simulink model "D_Latch"  (R2020a)
settings: Solver=VariableStepAuto  StartTime=0.0  StopTime=10.0  RelTol=1e-3
settings Model: Creator=ashwin  LastModifiedBy=ashwin

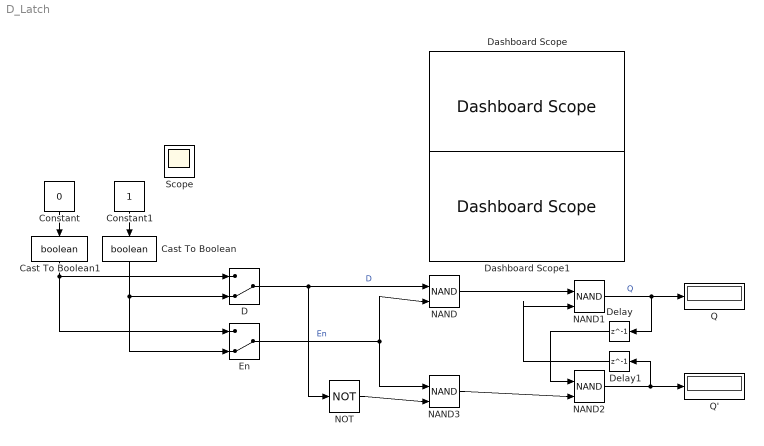
== system D_Latch ==
  Cast To Boolean : DataTypeConversion  OutDataTypeStr=boolean
  Cast To Boolean1 : DataTypeConversion  OutDataTypeStr=boolean
  Constant : Constant  Value=0
  Constant1 : Constant
  D : ManualSwitch  CurrentSetting=0
  Dashboard Scope : DashboardScope  Ymin=-0.5  Ymax=1.5
  Dashboard Scope1 : DashboardScope  Ymin=-0.5  Ymax=1.5
  Delay : Delay  DelayLength=1  InitialCondition=0
  Delay1 : Delay  DelayLength=1  InitialCondition=1
  En : ManualSwitch  CurrentSetting=0
  NAND{,1..3} (4 alike) : Logic  Operator=NAND  IconShape=distinctive  AllPortsSameDT=off  OutDataTypeStr=boolean
  NOT : Logic  Operator=NOT  IconShape=distinctive  AllPortsSameDT=off  OutDataTypeStr=boolean
  Q : Display
  Q' : Display
  Scope : Scope
  wires:
  D/1 -> NOT/1, NAND/1  "D"
  En/1 -> NAND/2, NAND3/1  "En"
  NAND/1 -> NAND1/1
  NAND3/1 -> NAND2/2
  NAND1/1 -> Delay/1, Q/1  "Q"
  NAND2/1 -> Delay1/1, Q'/1
  Constant/1 -> Cast To Boolean1/1
  Constant1/1 -> Cast To Boolean/1
  NOT/1 -> NAND3/2
  Delay/1 -> NAND2/1
  Delay1/1 -> NAND1/2
  Cast To Boolean/1 -> En/2, D/2
  Cast To Boolean1/1 -> D/1, En/1
